simulink model "MMG_Model"  (R2022a)
settings: Solver=VariableStepAuto  StartTime=0.0  StopTime=100  RelTol=1e-3
settings Model: Creator=Z0150218  LastModifiedBy=Z0150218

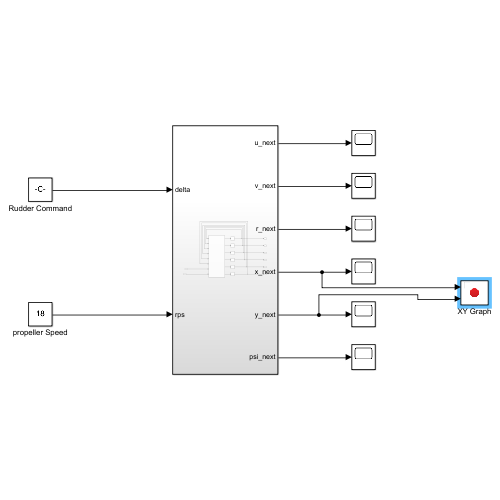
[thumbnail: Simulink's stored preview of the top-level diagram]
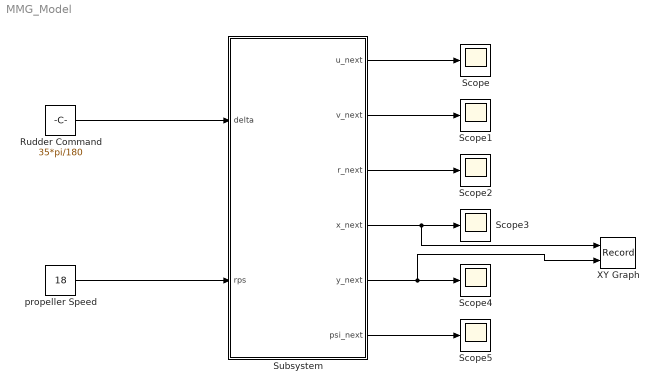
== system MMG_Model ==
  Rudder Command : Constant  Value=35*pi/180
  Scope{,1..5} (6 alike) : Scope
  Subsystem : Subsystem
  XY Graph : Record  FileSettingsInternal="{\"entries\":[{\"content\":{\"excelSettings\":{\"content\":{},\"type\":\"Streamout.ExcelSettings\"}},\"type\":\"Streamout.FileSettingStorage\",\"uuid\":\"59b6c840-506a-4456-8290-f92885f89b41\"}],\"packageUris\":[\"http://schema.mathworks.com/mf0/streamout_blocks/R2020a\"],\"version\":\"1.0\"}"  Layout=[1 1]  SignalsInternal="{\"entries\":[{\"content\":{\"signals\":[{\"content\":{\"blockPath\":[\"MMG_Model/XY Graph\"],\"channel\":[],\"dimensions\":[1],\"domain\":\"MMG_Model/XY Graph\",\"lineColor\":\"#a2142f\",\"plots\":[1],\"port\":1,\"sid\":[\"\"],\"signalID\":28,\"signalName\":\"Subsystem:4\"},\"type\":\"RecordBlkView.Signal\",\"uuid\":\"2fd87267-67ca-49b3-b818-3d1452393c92\"},{\"content\":{\"blockPath\":[\"MMG_Model/XY Graph\"],\"channel\":[],\"dimensions\":[1],\"domain\":\"MMG_Model/XY Graph\",\"lineColor\":\"#139fff\",\"plots\":[1],\"port\":2,\"sid\":[\"\"],\"signalID\":32,\"signalName\":\"Subsystem:5\"},\"type\":\"RecordBlkView.Signal\",\"uuid\":\"34f33422-a6e6-4da2-ada3-516180c28368\"}]},\"type\":\"RecordBlkView.InputSignals\",\"uuid\":\"e6691043-ef76-4adb-aa98-9ff712d68774\"}],\"packageUris\":[\"http://schema.mathworks.com/mf0/streamout_blocks/R2020a\"],\"version\":\"1.0\"}"  VisualizationBindings="{\"xyplotplugin\":{\"info\":[{\"series\":[{\"bindingParametersList\":[{\"parameter\":\"X-Axis\",\"signalID\":28,\"signalName\":\"Subsystem:4\"},{\"parameter\":\"Y-Axis\",\"signalID\":32,\"signalName\":\"Subsystem:5\"}],\"seriesID\":42964}],\"subplotID\":1}]}}"  CompatibilityTag=XY
  propeller Speed : Constant  Value=18
  wires:
  Rudder Command/1 -> Subsystem/1(delta)
  propeller Speed/1 -> Subsystem/2(rps)
  Subsystem/1(u_next) -> Scope/1
  Subsystem/2(v_next) -> Scope1/1
  Subsystem/3(r_next) -> Scope2/1
  Subsystem/4(x_next) -> XY Graph/1, Scope3/1
  Subsystem/5(y_next) -> XY Graph/2, Scope4/1
  Subsystem/6(psi_next) -> Scope5/1

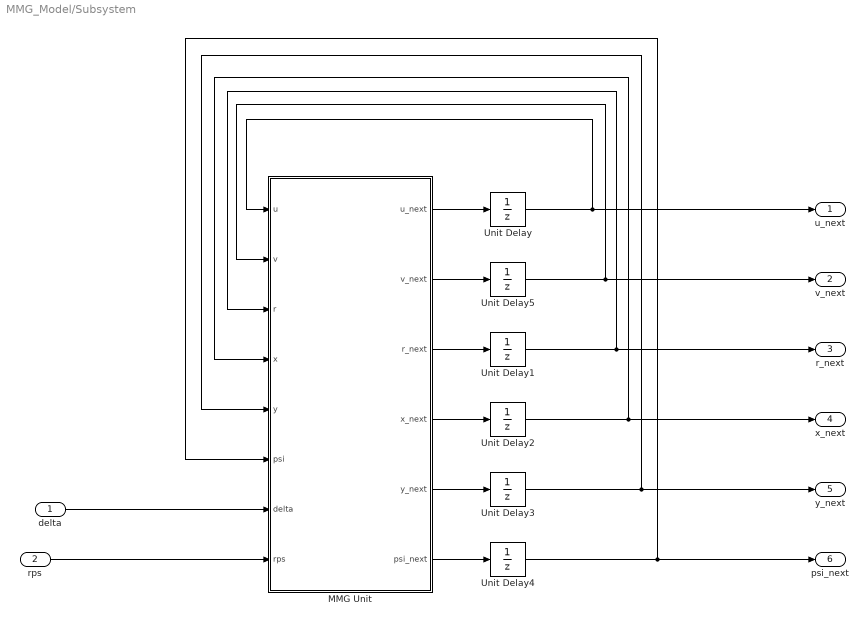
== system MMG_Model/Subsystem ==
  delta : Inport
  rps : Inport  Port=2
  MMG Unit : Subsystem
  Unit Delay : UnitDelay  InitialCondition=1.28  SampleTime=0.05  HasFrameUpgradeWarning=on
  Unit Delay{1..5} (5 alike) : UnitDelay  SampleTime=0.05  HasFrameUpgradeWarning=on
  u_next : Outport
  v_next : Outport  Port=2
  r_next : Outport  Port=3
  x_next : Outport  Port=4
  y_next : Outport  Port=5
  psi_next : Outport  Port=6
  wires:
  MMG Unit/4(x_next) -> Unit Delay2/1
  MMG Unit/6(psi_next) -> Unit Delay4/1
  MMG Unit/2(v_next) -> Unit Delay5/1
  Unit Delay/1 -> u_next/1, MMG Unit/1(u)
  Unit Delay4/1 -> psi_next/1, MMG Unit/6(psi)
  MMG Unit/1(u_next) -> Unit Delay/1
  MMG Unit/5(y_next) -> Unit Delay3/1
  MMG Unit/3(r_next) -> Unit Delay1/1
  Unit Delay3/1 -> y_next/1, MMG Unit/5(y)
  Unit Delay5/1 -> v_next/1, MMG Unit/2(v)
  Unit Delay1/1 -> r_next/1, MMG Unit/3(r)
  Unit Delay2/1 -> x_next/1, MMG Unit/4(x)
  delta/1 -> MMG Unit/7(delta)
  rps/1 -> MMG Unit/8(rps)

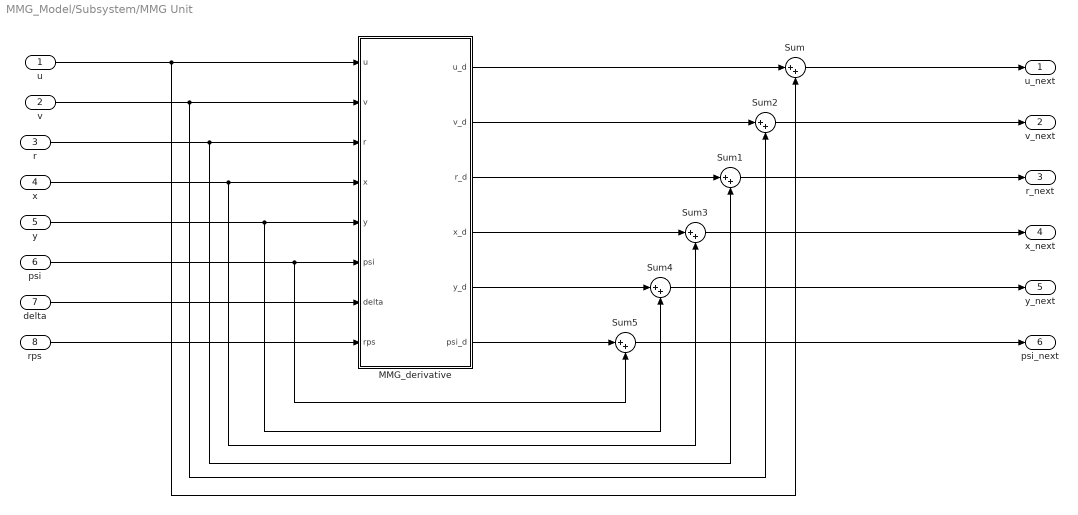
== system MMG_Model/Subsystem/MMG Unit ==
  u : Inport
  v : Inport  Port=2
  r : Inport  Port=3
  x : Inport  Port=4
  y : Inport  Port=5
  psi : Inport  Port=6
  delta : Inport  Port=7
  rps : Inport  Port=8
  MMG_derivative : MATLAB Function  TreatAsAtomicUnit=on
  Sum{,1..5} (6 alike) : Sum  Inputs=|++
  u_next : Outport
  v_next : Outport  Port=2
  r_next : Outport  Port=3
  x_next : Outport  Port=4
  y_next : Outport  Port=5
  psi_next : Outport  Port=6
  wires:
  MMG_derivative/2(v_d) -> Sum2/1
  MMG_derivative/1(u_d) -> Sum/1
  v/1 -> Sum2/2, MMG_derivative/2(v)
  psi/1 -> Sum5/2, MMG_derivative/6(psi)
  delta/1 -> MMG_derivative/7(delta)
  MMG_derivative/5(y_d) -> Sum4/1
  y/1 -> Sum4/2, MMG_derivative/5(y)
  r/1 -> Sum1/2, MMG_derivative/3(r)
  MMG_derivative/6(psi_d) -> Sum5/1
  u/1 -> Sum/2, MMG_derivative/1(u)
  Sum2/1 -> v_next/1
  MMG_derivative/3(r_d) -> Sum1/1
  MMG_derivative/4(x_d) -> Sum3/1
  x/1 -> Sum3/2, MMG_derivative/4(x)
  Sum5/1 -> psi_next/1
  Sum4/1 -> y_next/1
  Sum1/1 -> r_next/1
  Sum/1 -> u_next/1
  rps/1 -> MMG_derivative/8(rps)
  Sum3/1 -> x_next/1

== matlab function MMG_Model/Subsystem/MMG Unit/MMG_derivative ==
  data: u input; u_d output; v input; r input; x input; y input; psi input; delta input; rps input; v_d output; r_d output; x_d output; y_d output; psi_d output
function [u_d,v_d,r_d,x_d,y_d,psi_d] = MMG_Time_Derivative(u,v,r,x,y,psi,delta,rps)
%%%%%%%%%%%%%%%%%%%%%%%%%%%%%%%%%%%%%%%%%%%%%%
%%%%%%%%%% Assertion %%%%%%%%%%%
if u <= 0
    u = 0.00001;
end
if rps <= 0
    rps = 1;
end
%%%%%%%%%%%%%%%%%%%%%%%%%%%%%%%%%%%%%%%%%%%%%%
U             = sqrt((u^2)+(v^2));   % Resultant speed
beta          = atan(-v/u);        % Hull drift angle at midship
Np            = rps;                 % just for notation

%%%%%%%%%%%%%%%%%%%%%%%%%%%%%%%%%%%%%%%%%%%%%%
%%%%%% Kinematic Parameters of the ship %%%%%%
%%%%%%%%%%%%%%%%%%%%%%%%%%%%%%%%%%%%%%%%%%%%%%
Lpp     = 7;      % length between perpenticular
d       = 0.46;   % ship draft
xG      = 0.25;   % Longitudinal coordinate of center of gravity of ship
rho     = 1025;   % Water density
Volume  = 3.27;   % Displacement volume of ship
%%%%%%%%%%%%%%%%%%%%%%%%%%%%%%%%%%%%%%%%%%%%%%%%%%%%%
%%% Mass, Added Mass and Added Moment of inertia %%%%
%%%%%%%%%%%%%%%%%%%%%%%%%%%%%%%%%%%%%%%%%%%%%%%%%%%%%
mx          = 0.022;
my          = 0.223;
jz          = 0.011;
%%%%%%%%%% DiMensionalizing(dm) parameters %%%%%%%%%%
dm_force   = 0.5*rho*Lpp*d*(U^2);
dm_moment  = 0.5*rho*(Lpp^2)*d*(U^2);
dm_mass    = 0.5*rho*d*(Lpp^2);
dm_massMoI = 0.5*rho*d*(Lpp^4);
%%%%%%%%%% Dimensional mass %%%%%%%%%%%%%
mx      = mx*dm_mass;
my      = my*dm_mass;
jz      = jz*dm_massMoI;
m       = Volume*rho;
IzG     = m * ((0.25*Lpp)^2);  % Moment of inertia of ship around center of gravity
%%%%%%%%%%%%%%%%%%%%%%%%%%%%%%%%%%%%%%%%%%%%%%%%%%%%%%%
%%%%%%%%%%%% Governing Equation (Equation 4) %%%%%%%%%%
%%%%%%%%%%%%%%%%%%%%%%%%%%%%%%%%%%%%%%%%%%%%%%%%%%%%%%%

%%%%%%%%%% Mass Matrix %%%%%%%%%%%%%
M       = [(m+mx) 0 0;
            0 (m+my) m*xG;
            0 m*xG (jz+((xG^2)*m)+IzG)];

%%%%%%%%%%%%%%% LHS %%%%%%%%%%%%%%%%
LHS_r = [-(m+my)*v*r-xG*m*(r^2);
        (m+mx)*u*r;
        m*xG*u*r];

%%%%%%%%%%%%%%%%%%%%%%%%%%%%%%%%%%%%%%%%%%%%%%%%%%%%%%%
%%%%%%%%%%%  Hydrodynamic Force on Hull(F_hull) %%%%%%%
%%%%%%%%%%%%%%%%%%%%%%%%%%%%%%%%%%%%%%%%%%%%%%%%%%%%%%%

%%%%%% Non Dimensional Velocity and yaw %%%%%%%
v_ndm       = v/U;
r_ndm       = r*Lpp/U;
    
R0          = 0.022; % Ship resistance coefficient in straight moving
%%%%%% Non Dimensional Hydrodynamic Derivatives %%%%%
[X_vv, X_vr ,X_rr ,X_vvvv]             = deal(-0.04, 0.002, 0.011, 0.771);
[Y_v, Y_R, Y_vvv, Y_vvr, Y_vrr, Y_rrr] = deal(-0.315, 0.083, -1.607, 0.379, -0.391, 0.008);
[N_v, N_R, N_vvv, N_vvr, N_vrr, N_rrr] = deal(-0.137, -0.049, -0.03, -0.294, 0.055, -0.013);
%%%%%% Force and Moment %%%%%
X_hull      =  -R0 + (X_vv*(v_ndm^2)) + (X_vr*v_ndm*r_ndm) + (X_rr*(r_ndm^2)) + (X_vvvv*(v_ndm^4));
            
Y_hull      =  (Y_v*v_ndm) + (Y_R*r_ndm) + (Y_vvv*(v_ndm^3)) + (Y_vvr*(v_ndm^2)*r_ndm) + (Y_vrr*v_ndm*(r_ndm^2)) + (Y_rrr*(r_ndm^3));
            
N_hull      = (N_v*v_ndm) + (N_R*r_ndm) + (N_vvv*(v_ndm^3)) + (N_vvr*(v_ndm^2)*r_ndm) + (N_vrr*v_ndm*(r_ndm^2)) + (N_rrr*(r_ndm^3));
%%%%%%% Equation 6 %%%%%%%
X_hull = dm_force * X_hull;
Y_hull = dm_force * Y_hull;
N_hull = dm_moment* N_hull;
%%%%%%% Hull Force %%%%%%%
F_hull = [X_hull; Y_hull; N_hull];
%%%%%%%%%%%%%%%%%%%%%%%%%%%%%%%%%%%%%%%%%%%%%%%%%%%%%%%%%%%%
%%%%%%%%%%%% Propellar Force on Ship(F_propellar) %%%%%%%%%%
%%%%%%%%%%%%%%%%%%%%%%%%%%%%%%%%%%%%%%%%%%%%%%%%%%%%%%%%%%%%
tp          = 0.220;                        % Thrust deduction factor
Dp          = 0.216;                        % Propeller diameter
wp0         = 0.40;                         % Effective wake in straight moving
[k0,k1,k2]  = deal(0.2931, -0.2753, -0.1385);% 2nd order polynomial function coefficient
xP          = -0.48;                        % Longitudinal coordinate of propeller position
beta_P      = beta - (xP * r_ndm);          % geometrical inflow angle 

wp          =  wp0*exp(-4*(beta_P^2));      % Equation 12
Jp          =  u*(1-wp)/(Np*Dp);            % Equation 11
KT          =  k0 + k1*Jp + k2*(Jp^2);      % Equation 10
T           =  rho*(Np^2)*(Dp^4)*KT;        % Equation 9
X_propellar =  (1 - tp)*T;                  % Equation 8

%%%%%%%%% Propellar Force %%%%%%%%%%
F_propellar = [X_propellar; 0; 0];
%%%%%%%%%%%%%%%%%%%%%%%%%%%%%%%%%%%%%%%%%%%%%%%%%%%%%%%%%%%
%%%%%%%%%%%%%% Rudder Force on Ship(F_rudder)  %%%%%%%%%%%%
%%%%%%%%%%%%%%%%%%%%%%%%%%%%%%%%%%%%%%%%%%%%%%%%%%%%%%%%%%%     
%%%%%%% Equation 46 %%%%%%%%%%
epsilon    = 1.09;                   % Ratio of wake fraction
k          = 0.5;                    % An experimental constant for expressing uR
HR         = 0.345;                  % Rudder span length
eta        = Dp/HR;                  % Ratio of propeller diameter to rudderspan 
uP         = (1 - wp)*u;             % propeller inflow velocity

uR1   = sqrt(1 + ((8*KT)/(pi*(Jp^2))));
uR2   = (1 + k*(uR1 -1))^2;
uR    = epsilon * uP * sqrt( (eta*uR2) + (1-eta));

%%%%%%%%%%%%% Equation 23 %%%%%%%%%%%%%%%
lR          = -0.710;                        % Effective longitudinal coordinate
beta_R      =  beta -(lR*r_ndm);             % Effective inflow angle to rudder in maneuvering motions
if beta_R < 0
    gamma_r     = 0.396;                     % Flow straightening coefficient
else
    gamma_r     = 0.64;
end

vR    =  U * gamma_r * beta_R;

%%%%%%% Equation 19 %%%%%%%%
AR          = 0.0539;                    % Profile area of movable part of mariner rudder
f_alpha     = 2.747;                     % Rudder lift gradient coefficient
alpha_R     = delta - atan(vR/uR);       % Effective inflow angle to rudder
Ur          = sqrt((uR^2)+(vR^2));       % Resultant inflow velocity to rudder

F_normal = 0.5 * rho * AR * (Ur^2) * f_alpha * sin(alpha_R);

%%%%%%%%%%%% Equation 18 %%%%%%%%%%%%
tR         = 0.387;                      % Steering resistance deduction factor
aH         = 0.312;                      % Rudder force increase factor
xH         = -0.45* Lpp;                 % Longitudinal coordinate of acting point of the additional lateral force
xR         = -0.5 * Lpp;                 % Longitudinal coordinate of rudder position 

X_rudder =  -(1 - tR) * F_normal * sin(delta);
Y_rudder =  -(1 + aH) * F_normal * cos(delta);
N_rudder =  -(xR + (aH*xH)) * F_normal * cos(delta);

%%%%%%%%%% Rudder Force %%%%%%%%%%%
F_rudder = [X_rudder; Y_rudder; N_rudder];

%%%%%%%%%%%%%%%%%%%%%%%%%%%%%%%%%%%%%%%%%%%%%%%%%%%%%%%%
%%%%%%% Solution of Governing Equation (A.X = b)  %%%%%%
%%%%%%%%%%%%%%%%%%%%%%%%%%%%%%%%%%%%%%%%%%%%%%%%%%%%%%%%
b               = F_hull + F_propellar + F_rudder - LHS_r;

%%%%%%%%%% u_dot,v_dot,r_dot %%%%%%%%%%
X   = M\b;
%%%%%%%%%%%%%%%%%%%%%%%%%%%%%%%%%%%%%%%%%%%%%%%%%%%%%%%%
%%%%%%%%%%%%%%%%%%% Kinetics of the Ship  %%%%%%%%%%%%%%
%%%%%%%%%%%%%%%%%%%%%%%%%%%%%%%%%%%%%%%%%%%%%%%%%%%%%%%%%
%%%%%% Rotation Matrix %%%%%%%%%
R       =  [cos(psi) -sin(psi) 0; sin(psi) cos(psi)  0; 0  0 1];
%%%%%%%%% Velocity and Moment %%%%%%%%%%%
Vel_Mom = R*[u; v; r];

[u_d,v_d,r_d,x_d,y_d,psi_d] = deal(X(1),X(2),X(3),Vel_Mom(1),Vel_Mom(2),Vel_Mom(3));

end
